simulink library "DQN_Machines"  (R2023b)
settings: Solver=VariableStepAuto  StartTime=0.0  StopTime=10.0  RelTol=1e-3
undefined symbols (not defined in the file): DiscIntNeverNeededParam, N, SM, Ts
libraries: spsabctodq0Lib x2, spsdq0toabcLib x2
(part 5 of 5)

== system DQN_Machines/#BACKUP/DQN_Mac_V3/sin,cos ==
  theta : Inport
  Elementary Math : Trigonometry
  Elementary Math1 : Trigonometry  Operator=cos
  Mux3 : Mux  Inputs=2
  sin,cos : Outport  InitialOutput=0  VectorParamsAs1DForOutWhenUnconnected=off
  wires:
  theta/1 -> Elementary Math/1, Elementary Math1/1
  Elementary Math/1 -> Mux3/1
  Elementary Math1/1 -> Mux3/2
  Mux3/1 -> sin,cos/1

== system DQN_Machines/DQN_Mac_V1/Mechanical model1/Delay Prediction ==
  in : Inport
  F2 : Gain  Gain=2  SaturateOnIntegerOverflow=on  OutDataTypeStr=Inherit: Same as input  ParamDataTypeStr=Inherit: Same as input
  Sum1 : Sum  Inputs=+-  InputSameDT=on  SaturateOnIntegerOverflow=on  OutDataTypeStr=Inherit: Same as first input
  dw_delay : UnitDelay  InitialCondition=SMRD.dwo  SampleTime=SMRD.Ts  HasFrameUpgradeWarning=on
  dw_predict : UnitDelay  InitialCondition=SMRD.dwo  SampleTime=SMRD.Ts  HasFrameUpgradeWarning=on
  dw : Outport  VectorParamsAs1DForOutWhenUnconnected=off
  wires:
  dw_delay/1 -> dw_predict/1, F2/1
  in/1 -> dw_delay/1
  dw_predict/1 -> Sum1/2
  F2/1 -> Sum1/1
  Sum1/1 -> dw/1

== system DQN_Machines/#BACKUP/DQN_Mac_V1/Mechanical model/Delay Prediction ==
  in : Inport
  F2 : Gain  Gain=2  SaturateOnIntegerOverflow=on  OutDataTypeStr=Inherit: Same as input  ParamDataTypeStr=Inherit: Same as input
  Sum1 : Sum  Inputs=+-  InputSameDT=on  SaturateOnIntegerOverflow=on  OutDataTypeStr=Inherit: Same as first input
  dw_delay : UnitDelay  InitialCondition=SMRD.dwo  SampleTime=SMRD.Ts  HasFrameUpgradeWarning=on
  dw_predict : UnitDelay  InitialCondition=SMRD.dwo  SampleTime=SMRD.Ts  HasFrameUpgradeWarning=on
  dw : Outport  VectorParamsAs1DForOutWhenUnconnected=off
  wires:
  dw_delay/1 -> dw_predict/1, F2/1
  in/1 -> dw_delay/1
  dw_predict/1 -> Sum1/2
  F2/1 -> Sum1/1
  Sum1/1 -> dw/1

== system DQN_Machines/#BACKUP/DQN_Mac_V1_old/Mechanical model/Delay Prediction ==
  in : Inport
  F2 : Gain  Gain=2  SaturateOnIntegerOverflow=on  OutDataTypeStr=Inherit: Same as input  ParamDataTypeStr=Inherit: Same as input
  Sum1 : Sum  Inputs=+-  InputSameDT=on  SaturateOnIntegerOverflow=on  OutDataTypeStr=Inherit: Same as first input
  dw_delay : UnitDelay  InitialCondition=SMRD.dwo  SampleTime=SMRD.Ts  HasFrameUpgradeWarning=on
  dw_predict : UnitDelay  InitialCondition=SMRD.dwo  SampleTime=SMRD.Ts  HasFrameUpgradeWarning=on
  dw : Outport  VectorParamsAs1DForOutWhenUnconnected=off
  wires:
  dw_delay/1 -> dw_predict/1, F2/1
  in/1 -> dw_delay/1
  dw_predict/1 -> Sum1/2
  F2/1 -> Sum1/1
  Sum1/1 -> dw/1

== system DQN_Machines/#BACKUP/DQN_Mac_V2/Mechanical model/Delay Prediction ==
  in : Inport
  F2 : Gain  Gain=2  SaturateOnIntegerOverflow=on  OutDataTypeStr=Inherit: Same as input  ParamDataTypeStr=Inherit: Same as input
  Sum1 : Sum  Inputs=+-  InputSameDT=on  SaturateOnIntegerOverflow=on  OutDataTypeStr=Inherit: Same as first input
  dw_delay : UnitDelay  InitialCondition=SMRD.dwo  SampleTime=SMRD.Ts  HasFrameUpgradeWarning=on
  dw_predict : UnitDelay  InitialCondition=SMRD.dwo  SampleTime=SMRD.Ts  HasFrameUpgradeWarning=on
  dw : Outport  VectorParamsAs1DForOutWhenUnconnected=off
  wires:
  Sum1/1 -> dw/1
  F2/1 -> Sum1/1
  dw_predict/1 -> Sum1/2
  in/1 -> dw_delay/1
  dw_delay/1 -> F2/1, dw_predict/1

== system DQN_Machines/#BACKUP/DQN_Mac_V2_untested/Mechanical model/Delay Prediction ==
  in : Inport
  F2 : Gain  Gain=2  SaturateOnIntegerOverflow=on  OutDataTypeStr=Inherit: Same as input  ParamDataTypeStr=Inherit: Same as input
  Sum1 : Sum  Inputs=+-  InputSameDT=on  SaturateOnIntegerOverflow=on  OutDataTypeStr=Inherit: Same as first input
  dw_delay : UnitDelay  InitialCondition=SMRD.dwo  SampleTime=SMRD.Ts  HasFrameUpgradeWarning=on
  dw_predict : UnitDelay  InitialCondition=SMRD.dwo  SampleTime=SMRD.Ts  HasFrameUpgradeWarning=on
  dw : Outport  VectorParamsAs1DForOutWhenUnconnected=off
  wires:
  dw_delay/1 -> dw_predict/1, F2/1
  in/1 -> dw_delay/1
  dw_predict/1 -> Sum1/2
  F2/1 -> Sum1/1
  Sum1/1 -> dw/1

== system DQN_Machines/#BACKUP/DQN_Mac_V3/Mechanical model1/Delay Prediction ==
  in : Inport
  F2 : Gain  Gain=2  SaturateOnIntegerOverflow=on  OutDataTypeStr=Inherit: Same as input  ParamDataTypeStr=Inherit: Same as input
  Sum1 : Sum  Inputs=+-  InputSameDT=on  SaturateOnIntegerOverflow=on  OutDataTypeStr=Inherit: Same as first input
  dw_delay : UnitDelay  InitialCondition=SMRD.dwo  SampleTime=SMRD.Ts  HasFrameUpgradeWarning=on
  dw_predict : UnitDelay  InitialCondition=SMRD.dwo  SampleTime=SMRD.Ts  HasFrameUpgradeWarning=on
  dw : Outport  VectorParamsAs1DForOutWhenUnconnected=off
  wires:
  dw_delay/1 -> dw_predict/1, F2/1
  in/1 -> dw_delay/1
  dw_predict/1 -> Sum1/2
  F2/1 -> Sum1/1
  Sum1/1 -> dw/1

== matlab function DQN_Machines/#BACKUP/DQN_Mac_V2/MATLAB Function1 ==
  data: Vdq_vec input; Vs_c output; N parameter
function Vs_c   = fDQN012c(Vdq_vec, N)


    Vs_c  = complex(zeros(3, N+1));
    % Vr1_c = complex(zeros(3, N+1));
    % Vr2_c = complex(zeros(3, N+1));

    Vs_c(1,2)  = Vdq_vec(1) + 1i*Vdq_vec(2);
    % Vr1_c(1,2) = Vdq_vec(3) + 1i*Vdq_vec(4);
    % Vr2_c(1,2) = Vdq_vec(5) + 1i*Vdq_vec(6);



end

== matlab function DQN_Machines/#BACKUP/DQN_Mac_V2_untested/MATLAB Function1 ==
  data: Vdq_vec input; Vs_c output; N parameter
function Vs_c   = fDQN012c(Vdq_vec, N)


    Vs_c  = complex(zeros(3, N+1));
    % Vr1_c = complex(zeros(3, N+1));
    % Vr2_c = complex(zeros(3, N+1));

    Vs_c(1,2)  = Vdq_vec(1) + 1i*Vdq_vec(2);
    % Vr1_c(1,2) = Vdq_vec(3) + 1i*Vdq_vec(4);
    % Vr2_c(1,2) = Vdq_vec(5) + 1i*Vdq_vec(6);



end

== matlab function DQN_Machines/#BACKUP/DQN_Mac_V3/MATLAB Function2 ==
  data: Vdq_vec input; Vs_c output; N parameter
function Vs_c   = fDQN012c(Vdq_vec, N)


    Vs_c  = complex(zeros(3, N+1));
    % Vr1_c = complex(zeros(3, N+1));
    % Vr2_c = complex(zeros(3, N+1));

    Vs_c(1,2)  = Vdq_vec(1) + 1i*Vdq_vec(2);
    % Vr1_c(1,2) = Vdq_vec(3) + 1i*Vdq_vec(4);
    % Vr2_c(1,2) = Vdq_vec(5) + 1i*Vdq_vec(6);



end

== matlab function DQN_Machines/#BACKUP/DQN_Mac_V1/MATLAB Function1 ==
  data: Vdq_vec input; Vs_c output; N parameter
function Vs_c   = fDQN012c(Vdq_vec, N)


    Vs_c  = complex(zeros(3, N+1));
    % Vr1_c = complex(zeros(3, N+1));
    % Vr2_c = complex(zeros(3, N+1));

    Vs_c(1,2)  = Vdq_vec(1) + 1i*Vdq_vec(2);
    % Vr1_c(1,2) = Vdq_vec(3) + 1i*Vdq_vec(4);
    % Vr2_c(1,2) = Vdq_vec(5) + 1i*Vdq_vec(6);



end

== matlab function DQN_Machines/DQN_Mac_V1/MATLAB Function2 ==
  data: Vdq_vec input; Vs_c output; N parameter
function Vs_c   = fDQN012c(Vdq_vec, N)


    Vs_c  = complex(zeros(3, N+1));
    % Vr1_c = complex(zeros(3, N+1));
    % Vr2_c = complex(zeros(3, N+1));

    Vs_c(1,2)  = Vdq_vec(1) + 1i*Vdq_vec(2);
    % Vr1_c(1,2) = Vdq_vec(3) + 1i*Vdq_vec(4);
    % Vr2_c(1,2) = Vdq_vec(5) + 1i*Vdq_vec(6);



end

== matlab function DQN_Machines/#BACKUP/DQN_Mac_V1_old/MATLAB Function1 ==
  data: Vdq_vec input; Vs_c output; N parameter
function Vs_c   = fDQN012c(Vdq_vec, N)


    Vs_c  = complex(zeros(3, N+1));
    % Vr1_c = complex(zeros(3, N+1));
    % Vr2_c = complex(zeros(3, N+1));

    Vs_c(1,2)  = Vdq_vec(1) + 1i*Vdq_vec(2);
    % Vr1_c(1,2) = Vdq_vec(3) + 1i*Vdq_vec(4);
    % Vr2_c(1,2) = Vdq_vec(5) + 1i*Vdq_vec(6);



end
